simulink model "Day12"  (R2024b)
settings: Solver=VariableStepAuto  StartTime=0.0  StopTime=10.0  RelTol=1e-3
settings Model: Creator=jun_mac  LastModifiedBy=jun_mac

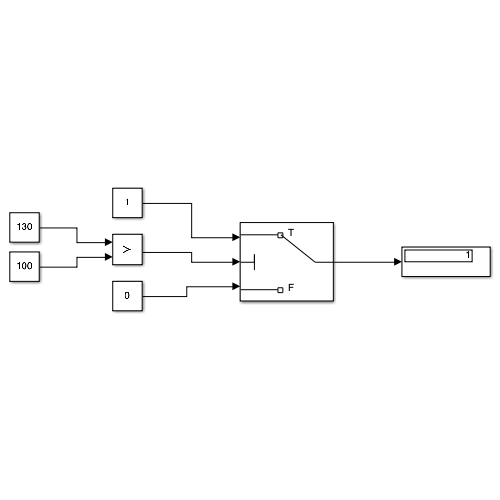
[thumbnail: Simulink's stored preview of the top-level diagram]
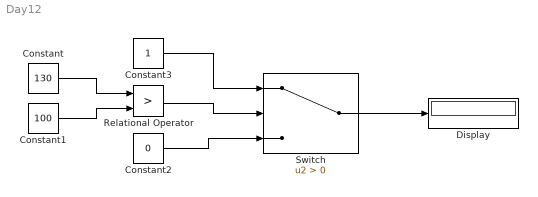
== system Day12 ==
  Constant : Constant  Value=130
  Constant1 : Constant  Value=100
  Constant2 : Constant  Value=0
  Constant3 : Constant
  Display : Display
  Relational Operator : RelationalOperator  Operator=>  OutDataTypeStr=boolean  RndMeth=Simplest  InputSameDT=off
  Switch : Switch  Criteria=u2 > Threshold  SaturateOnIntegerOverflow=off  InputSameDT=off
  wires:
  Constant/1 -> Relational Operator/1
  Switch/1 -> Display/1
  Constant2/1 -> Switch/3
  Relational Operator/1 -> Switch/2
  Constant3/1 -> Switch/1
  Constant1/1 -> Relational Operator/2
